simulink model "InteriorPMSMFieldOrientedControl1"  (R2024a)
settings: Solver=FixedStepDiscrete  StartTime=0.0  StopTime=2  RelTol=1e-3  EnableMultiTasking=on
PreLoadFcn:
  | InteriorPMSMFieldOrientedControlData_Lafae
InitFcn:
  | InteriorPMSMFieldOrientedControlData_Lafae
values from neighbouring files (symbols this model uses):
  F = 0.002    [InteriorPMSMFieldOrientedControlData_Lafae.m]
  Fsw = 8000    [InteriorPMSMFieldOrientedControlData_Lafae.m]
  J = 0.09    [InteriorPMSMFieldOrientedControlData_Lafae.m]
  Ki_Ireg = (Ki_Id + Ki_Iq)/2    (= 650)    [InteriorPMSMFieldOrientedControlData_Lafae.m]
  Ki_wreg = (alpha_s/(2*eta))^2*J    [InteriorPMSMFieldOrientedControlData_Lafae.m]
  Kp_Ireg = (Kp_Id + Kp_Iq)/2    (= 182.7)    [InteriorPMSMFieldOrientedControlData_Lafae.m]
  Kp_wreg = alpha_s * J    [InteriorPMSMFieldOrientedControlData_Lafae.m]
  lambda = 0.1757    [InteriorPMSMFieldOrientedControlData_Lafae.m]
  Ld = 1.597e-3    (= 0.001597)    [InteriorPMSMFieldOrientedControlData_Lafae.m]
  Ld_var = 0.9*1.597e-3    (= 0.0014373)    [InteriorPMSMFieldOrientedControlData_Lafae.m]
  Limit_Ireg = Vdc_nom/sqrt(3)    [InteriorPMSMFieldOrientedControlData_Lafae.m]
  Limit_wreg = Tnom    (= 400)    [InteriorPMSMFieldOrientedControlData_Lafae.m]
  Lq = 2.057e-3    (= 0.002057)    [InteriorPMSMFieldOrientedControlData_Lafae.m]
  Lq_var = 0.9*2.057e-3    (= 0.0018513)    [InteriorPMSMFieldOrientedControlData_Lafae.m]
  p = 4    [InteriorPMSMFieldOrientedControlData_Lafae.m]
  rpm_data = [0 1200 2000 3000 4000 5000 6000]    [InteriorPMSMFieldOrientedControlData_Lafae.m]
  Rs = 6.5e-3    (= 0.0065)    [InteriorPMSMFieldOrientedControlData_Lafae.m]
  Tmax_data = [400 400 225 150 100 80 70]    [InteriorPMSMFieldOrientedControlData_Lafae.m]
  Tnom = 400    [InteriorPMSMFieldOrientedControlData_Lafae.m]
  Ts = 10e-6    (= 1e-05)    [InteriorPMSMFieldOrientedControlData_Lafae.m]
  Vdc_nom = 550    [InteriorPMSMFieldOrientedControlData_Lafae.m]
  wmax = 6000    [InteriorPMSMFieldOrientedControlData_Lafae.m]
undefined symbols (not defined in the file or in its folder): DiscIntNeverNeededParam, gcbh, sps_rtmsupport
libraries: simulink x11, spsSecondOrderFilterLib x6, spsStairGeneratorLib x6, spsPermanentMagnetSynchronousMachineLib x1, spsDCVoltageSourceLib x1, spsdq0toabcLib x1, spsabctodq0Lib x1, spsPowerdq0InstantaneousLib x1, spsThreePhaseVIMeasurementLib x1, spsTwoLevelConverterLib x1, spspowerguiLib x1
settings Model: SimulationMode=accelerator  Creator=The MathWorks, Inc.  LastModifiedBy=luansantos
settings SolverCC: AlgebraicLoopSolver=TrustRegion
settings DataIOCC: SaveOutput=off  SignalLogging=off  DSMLogging=off  SaveTime=off  ReturnWorkspaceOutputs=off
settings DebuggingCC: UnconnectedInputMsg=warning  UnconnectedOutputMsg=warning  UnconnectedLineMsg=warning
settings ModelReferenceCC: EnableRefExpFcnMdlSchedulingChecks=on
settings RTWCC: GPUComputeCapability=3.5  DLArmComputeVersion=19.05

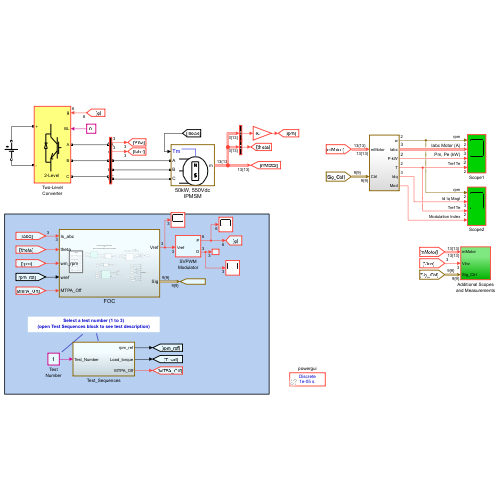
[thumbnail: Simulink's stored preview of the top-level diagram]
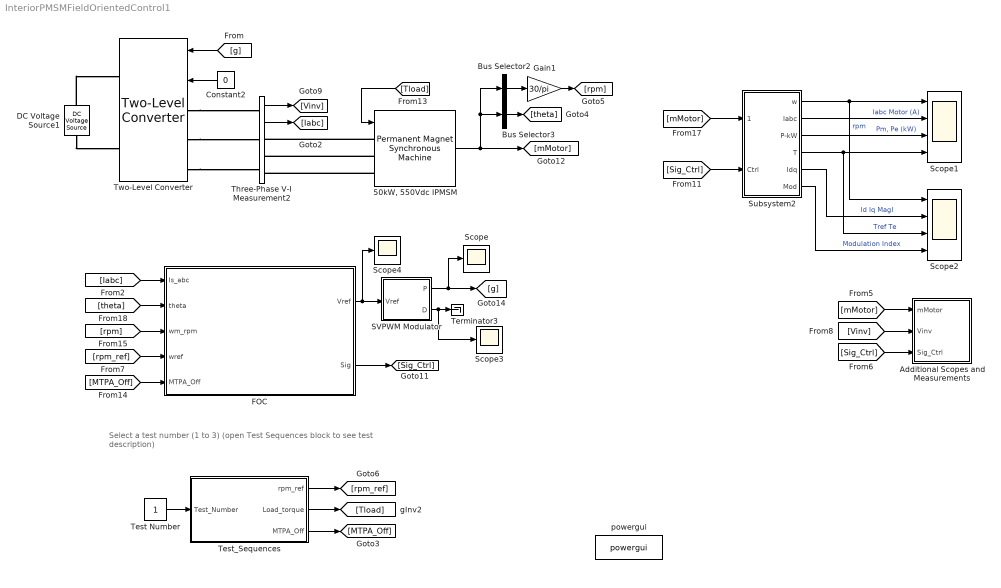
== system InteriorPMSMFieldOrientedControl1 ==
  note: Select a test number (1 to 3)
      | (open Test Sequences block to see test description)
  "50kW, 550Vdc IPMSM" : spsPermanentMagnetSynchronousMachineLib/Permanent Magnet Synchronous Machine  NbPhases=3  FluxDistribution=Sinusoidal  RotorType=Salient-pole  MechanicalLoad=Torque Tm  PresetModel=No  ShowDetailedParameters=on  MeasurementBus=off  Resistance=Rs  Inductance=8.5e-3  dqInductances=[Ld_var, Lq_var]  La=0.005/2  MachineConstant=Flux linkage established by magnets (V.s)  Flux=lambda_var  VoltageCst=127.4738  TorqueCst=1.0542  Flat=120  Mechanical=[J F p 0]  PolePairs=4  InitialConditions=[0,0, 0,0]  InitialConditions5ph=[0 0 0 0 0 0]  RefAngle=90 degrees behind phase A axis (modified Park)  IterativeDiscreteModel=Trapezoidal robust  TsBlock=Ts  TsPowergui=0
  Additional Scopes and Measurements : Subsystem
  Bus Selector2 : BusSelector  OutputSignals=Rotor speed wm (rad/s)  OutputAsBus=on
  Bus Selector3 : BusSelector  OutputSignals=Rotor angle thetam (rad)  OutputAsBus=on
  Constant2 : Constant  Value=0
  DC Voltage Source1 : spsDCVoltageSourceLib/DC Voltage Source  Amplitude=Vdc_nom  Measurements=None
  FOC : Subsystem
  Gain1 : Gain  Gain=30/pi
  SVPWM Modulator : Subsystem  DialogController=POWERSYS.PowerSysDialog  LoadFcn=sps_rtmsupport('LoadFcn', gcbh);  StartFcn=sps_rtmsupport('StartFcn', gcbh);  StopFcn=sps_rtmsupport('StopFcn', gcbh);  mask(Unified PWM Modulator for a 2-level, 3-phase converter){PWMmethod=Space Vector PWM (SVPWM) with pulse averaging, Fsw=Fsw, Ts=Ts}
      mask prompts: PWMmethod "PWM method"; Fsw "Switching frequency (Hz):"; Ts "Sample time (s):"
      mask help:
      | Generate pulses for PWM-controlled two-level, three-phase power electronics converter with pulse averaging capability.
      |
      | The pulses generation can be perform using one of the following Pulse-Width Modulation (PWM) methods:
      | 1. Sinusoidal PWM (SPWM)
      | 2. Sinusoidal PWM (SPWM) with pulse averaging
      | 3. Space Vector PWM (SVPWM)
      | 4. Space Vector PWM (SVPWM) with pulse averaging
      | 5. 30 degrees discontinuous PWM
      |
      | When a PWM method with pulse averaging is selected, the output pulses are averaged over one sample time. (Pulses value will range from 0 to 1)
      mask init:
      | switch PWMmethod
      |     case 1 % SPWM
      |         ZeroOrderHold_Ts=-1;
      |         Pavg=0;
      |     case 2 % SPWM with pulse averaging
      |         ZeroOrderHold_Ts=-1;
      |         Pavg=1;
      |     case 3  % SVPWM
      |         ZeroOrderHold_Ts=-1;
      |         Pavg=0;
      |     case 4  % SVPWM with pulse averaging
      |         ZeroOrderHold_Ts=-1;
      |         Pavg=1;
      |     case 5  % 30 degrees discontinuous PWM
      |         ZeroOrderHold_Ts=1/Fsw/2;
      |         Pavg=0;
      | end
      settings: CopyFcn=sps_rtmsupport('CopyFcn', gcbh);  DeleteFcn=sps_rtmsupport('DeleteFcn', gcbh);  UndoDeleteFcn=sps_rtmsupport('UndoDeleteFcn', gcbh);  ModelCloseFcn=sps_rtmsupport('ModelCloseFcn', gcbh);  PreSaveFcn=sps_rtmsupport('PreSaveFcn', gcbh);  PostSaveFcn=sps_rtmsupport('PostSaveFcn', gcbh);  NameChangeFcn=sps_rtmsupport('NameChangeFcn', gcbh);  PreCopyFcn=sps_rtmsupport('PreCopyFcn', gcbh);  OpenFcn=sps_rtmsupport('OpenFcn', gcbh, [1]);  CloseFcn=sps_rtmsupport('CloseFcn', gcbh);  PreDeleteFcn=sps_rtmsupport('PreDeleteFcn', gcbh);
      mask TypeOptions PWMmethod: Sinusoidal PWM (SPWM) | Sinusoidal PWM (SPWM) wirh pulse averaging | Space Vector PWM (SVPWM) | Space Vector PWM (SVPWM) with pulse averaging | 30 degrees discontinuous PWM
  Scope : Scope
  Scope1 : Scope  NumInputPorts=4
  Scope2 : Scope  NumInputPorts=4
  Scope3 : Scope
  Scope4 : Scope
  Subsystem2 : Subsystem
  Terminator3 : Terminator
  Test Number : Constant
  Test_Sequences : Subsystem
  Three-Phase V-I Measurement2 : spsThreePhaseVIMeasurementLib/Three-Phase V-I Measurement  VoltageMeasurement=phase-to-phase  SetLabelV=off  LabelV=Vabc  Vpu=off  VpuLL=off  CurrentMeasurement=yes  SetLabelI=off  LabelI=Iabc  Ipu=off  Pbase=100e6  Vbase=500e3  OutputType=Complex  PhasorSimulation=off  PSBequivalent=0
  Two-Level Converter : spsTwoLevelConverterLib/Two-Level Converter  ModelType=Switching function  Ron=1e-3  Rs=1e6  Cs=inf  Vforward=[0,0]  Ron_Diode=1e-3  Rs_Diode=1e6  Cs_Diode=inf  Vf_Diode=0  Rs_CurrentSource=inf  Ron_ACsource=1e-3
  powergui : spspowerguiLib/powergui  SimulationMode=Discrete  SampleTime=Ts  frequency=60  Iterations=50  frequencyindice=0  Pbase=100e6  ErrMax=1e-4  UnitsV=kV  UnitsW=MW  buscounter=0  FunctionMessages=off  echomessages=off  EnableUseOfTLC=off  CurrentSourceSwitches=off  DisableSnubberDevices=off  DisableRonSwitches=off  DisableVfSwitches=off  DisplayEquations=off  AutomaticDiscreteSolvers=off  SolverType=Tustin  Interpol=off  ExternalGateDelay=off  methode=off  Ts=0  x0status=blocks  SPID=off  SwTol=0  HookPort=off  NonlinearTolerance=1e-4  nMaxIteration=100  ContinueOnMaxIteration=off  RestoreLinks=warning  ResistiveCurrentMeasurement=off  Frange=[0:2:500]  Ylog=off  Xlog=on  ShowGrid=off  save=off  variable=ZData  structure=ScopeData3  ZoomFFT=off  StartTime=0.95  cycles=1  DisplayStyle=1  fundamental=166.67  FreqAxis=off  MaxFrequency=20000  frequencyindicesteady=1  RmsSteady=1  display=off
  wires:
  [Iabc] -> FOC/1(Is_abc)
  Gain1/1 -> [rpm]
  "50kW, 550Vdc IPMSM"/1 -> [mMotor], Bus Selector3/1, Bus Selector2/1
  Test Number/1 -> Test_Sequences/1(Test_Number)
  Test_Sequences/2(Load_torque) -> [Tload]
  [MTPA_Off] -> FOC/5(MTPA_Off)
  SVPWM Modulator/1(P) -> Scope/1, [g]
  [theta] -> FOC/2(theta)
  Constant2/1 -> Two-Level Converter/2
  FOC/2(Sig) -> [Sig_Ctrl]
  Test_Sequences/1(rpm_ref) -> [rpm_ref]
  [mMotor] -> Subsystem2/1(mMotor)
  [rpm] -> FOC/3(wm_rpm)
  SVPWM Modulator/2(D) -> Scope3/1, Terminator3/1
  Subsystem2/3(P-kW) -> Scope1/3  "Pm, Pe (kW)"
  Bus Selector2/1 -> Gain1/1
  FOC/1(Vref) -> Scope4/1, SVPWM Modulator/1(Vref)
  [rpm_ref] -> FOC/4(wref)
  Three-Phase V-I Measurement2/2 -> [Iabc]
  [Sig_Ctrl] -> Subsystem2/2(Ctrl)
  Three-Phase V-I Measurement2/1 -> [Vinv]
  Bus Selector3/1 -> [theta]
  [g] -> Two-Level Converter/1
  Subsystem2/2(Iabc) -> Scope1/2  "Iabc Motor (A)"
  Test_Sequences/3(MTPA_Off) -> [MTPA_Off]
  Subsystem2/1(w) -> Scope1/1, Scope2/1  "rpm"
  Subsystem2/5(Idq) -> Scope2/2  "Id Iq MagI"
  Subsystem2/4(T) -> Scope1/4, Scope2/3  "Tref Te"
  [Vinv] -> Additional Scopes and Measurements/2(Vinv)
  [mMotor] -> Additional Scopes and Measurements/1(mMotor)
  [Sig_Ctrl] -> Additional Scopes and Measurements/3(Sig_Ctrl)
  Subsystem2/6(Mod) -> Scope2/4  "Modulation Index"
  [Tload] -> "50kW, 550Vdc IPMSM"/1
  connections:
  DC Voltage Source1/LConn1 -- Two-Level Converter/RConn2
  Two-Level Converter/LConn2 -- Three-Phase V-I Measurement2/LConn2
  Two-Level Converter/LConn1 -- Three-Phase V-I Measurement2/LConn1
  DC Voltage Source1/RConn1 -- Two-Level Converter/RConn1
  "50kW, 550Vdc IPMSM"/LConn2 -- Three-Phase V-I Measurement2/RConn2
  Two-Level Converter/LConn3 -- Three-Phase V-I Measurement2/LConn3
  "50kW, 550Vdc IPMSM"/LConn1 -- Three-Phase V-I Measurement2/RConn1
  "50kW, 550Vdc IPMSM"/LConn3 -- Three-Phase V-I Measurement2/RConn3

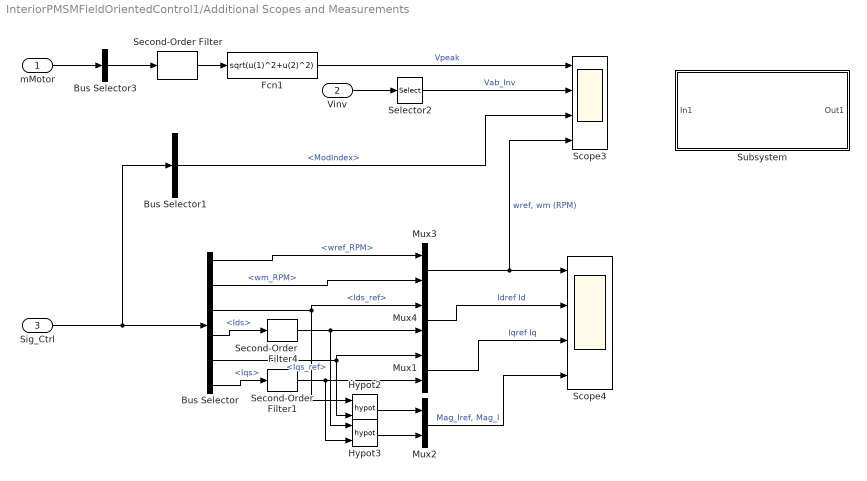
== system InteriorPMSMFieldOrientedControl1/Additional Scopes and Measurements ==
  mMotor : Inport
  Vinv : Inport  Port=2
  Sig_Ctrl : Inport  Port=3
  Bus Selector : BusSelector  OutputSignals=wref_RPM,wm_RPM,Ids_ref,Ids,Iqs_ref,Iqs
  Bus Selector1 : BusSelector  OutputSignals=ModIndex
  Bus Selector3 : BusSelector  OutputSignals=Stator voltage Vs_d (V),Stator voltage Vs_q (V)  OutputAsBus=on
  Fcn1 : Fcn  Expr=sqrt(u(1)^2+u(2)^2)
  Hypot2 : Math  Operator=hypot
  Hypot3 : Math  Operator=hypot
  Mux{1..4} (4 alike) : Mux  Inputs=2
  Scope3 : Scope  NumInputPorts=4
  Scope4 : Scope  NumInputPorts=4
  Second-Order Filter : spsSecondOrderFilterLib/Second-Order Filter  FilterType=Lowpass  Fo=120  Zeta=1  Ts=Ts  Initialize=off  Vac_Init="[0,  0,  60]"  Vdc_Init=0  PlotResponse=off  FreqRange=[0, 500, 1]
  Second-Order Filter1 : spsSecondOrderFilterLib/Second-Order Filter  FilterType=Lowpass  Fo=80  Zeta=1  Ts=Ts  Initialize=off  Vac_Init="[0,  0,  60]"  Vdc_Init=0  PlotResponse=off  FreqRange=[0, 500, 1]
  Second-Order Filter4 : spsSecondOrderFilterLib/Second-Order Filter  FilterType=Lowpass  Fo=80  Zeta=1  Ts=Ts  Initialize=off  Vac_Init="[0,  0,  60]"  Vdc_Init=0  PlotResponse=off  FreqRange=[0, 500, 1]
  Selector2 : Selector  InputPortWidth=3  IndexOptions=Index vector (dialog)  Indices=1  OutputSizes=1
  Subsystem : Subsystem
  wires:
  Bus Selector3/1 -> Second-Order Filter/1
  mMotor/1 -> Bus Selector3/1
  Second-Order Filter/1 -> Fcn1/1
  Bus Selector1/1 -> Scope3/3  "<ModIndex>"
  Mux2/1 -> Scope4/4  "Mag_Iref, Mag_I"
  Mux1/1 -> Scope4/3  "Iqref Iq"
  Mux4/1 -> Scope4/2  "Idref Id"
  Mux3/1 -> Scope4/1, Scope3/4  "wref, wm (RPM)"
  Bus Selector/2 -> Mux3/2  "<wm_RPM>"
  Bus Selector/1 -> Mux3/1  "<wref_RPM>"
  Hypot3/1 -> Mux2/2
  Hypot2/1 -> Mux2/1
  Second-Order Filter1/1 -> Mux1/2, Hypot3/2
  Second-Order Filter4/1 -> Mux4/2, Hypot3/1
  Bus Selector/6 -> Second-Order Filter1/1  "<Iqs>"
  Bus Selector/5 -> Hypot2/2, Mux1/1  "<Iqs_ref>"
  Bus Selector/4 -> Second-Order Filter4/1  "<Ids>"
  Bus Selector/3 -> Hypot2/1, Mux4/1  "<Ids_ref>"
  Sig_Ctrl/1 -> Bus Selector/1, Bus Selector1/1
  Vinv/1 -> Selector2/1
  Fcn1/1 -> Scope3/1  "Vpeak"
  Selector2/1 -> Scope3/2  "Vab_Inv"

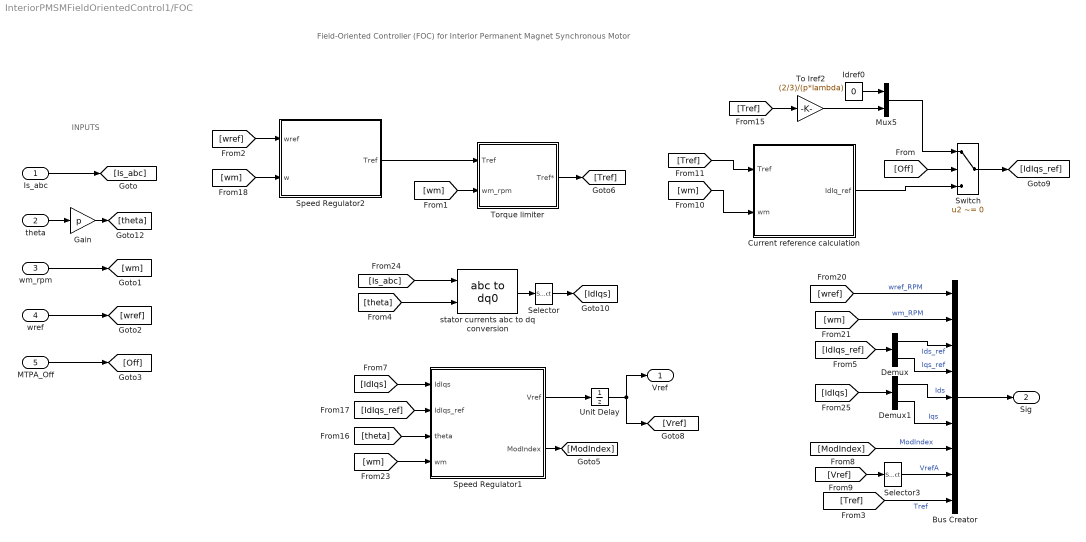
== system InteriorPMSMFieldOrientedControl1/FOC ==
  note: INPUTS
  note: Field-Oriented Controller (FOC)
      | for
      | Interior Permanent Magnet Synchronous Motor
  Is_abc : Inport  PortDimensions=3
  theta : Inport  Port=2  PortDimensions=1
  wm_rpm : Inport  Port=3  PortDimensions=1
  wref : Inport  Port=4  PortDimensions=1
  MTPA_Off : Inport  Port=5  PortDimensions=1
  Bus Creator : BusCreator  Inputs=9
  Current reference calculation : Subsystem  mask(Current reference generation){p=p, LdLq=[Ld, Lq], lambda=lambda, Ts=Ts}
      mask prompts: p "Motor pairs of poles"; LdLq "Inductances [ Ld(H) Lq(H) ]:"; lambda "Flux linkage established by magnets (V.s)"; Ts "Sampling time (s)"
      mask init:
      | Ld=LdLq(1);
      | Lq=LdLq(2);
      | ib = lambda/(Lq-Ld);
      | Teb = 3/2*p*lambda*ib;
      | lam = lambda;
      | ib = lam/(Lq-Ld);
      | iqn = 0:0.01:3;
      | ten = iqn/2.*(sqrt(4*iqn.*iqn+1)+1);
  Demux : Demux  Outputs=2
  Demux1 : Demux  Outputs=2
  Gain : Gain  Gain=p
  Idref0 : Constant  Value=0
  Mux5 : Mux  Inputs=2
  Selector : Selector  InputPortWidth=3  IndexOptions=Index vector (dialog)  Indices=[1 2]  OutputSizes=1
  Selector3 : Selector  InputPortWidth=3  IndexOptions=Index vector (dialog)  Indices=1  OutputSizes=1
  Speed Regulator1 : Subsystem  DialogController=POWERSYS.PowerSysDialog  mask(dq Current Regulators){Kp=Kp_Ireg, Ki=Ki_Ireg, Limits=Limit_Ireg, Init=0, Ts=Ts}
      mask prompts: Kp "Proportional gain (Kp):"; Ki "Integral gain (Ki):"; Limits "Output limits"; Init "Output initial value:"; Ts "Sample time:"
      mask help: This block implements dq currents regulator using anti-windup PI controllers and feedforward calculation.
      mask Display: disp('Current\nRegulators');
  Speed Regulator2 : Subsystem  DialogController=POWERSYS.PowerSysDialog  mask(Speed Regulator){Kp=Kp_wreg, Ki=Ki_wreg, Limit_wreg=Limit_wreg, Init=0, Ts=Ts}
      mask prompts: Kp "Proportional gain (Kp):"; Ki "Integral gain (Ki):"; Limit_wreg "Output limits"; Init "Output initial value:"; Ts "Sample time:"
      mask help: This block implements a speed regulator using an ant-windup PI controller.
      mask Display: disp('Speed\nRegulator');
  Switch : Switch  Criteria=u2 ~= 0  SaturateOnIntegerOverflow=off  InputSameDT=off
  To Iref2 : Gain  Gain=(2/3)/(p*lambda)
  Torque limiter : Subsystem
      mask Display: plot([0;1800;2000;2500;3000;3500], [1;1;0.90*1;0.72*1;0.6*1;0.51*1])
  Unit Delay : UnitDelay  SampleTime=-1  HasFrameUpgradeWarning=on
  stator currents abc to dq conversion : spsabctodq0Lib/abc to dq0  Alignment=90 degrees behind phase A axis
  Vref : Outport  PortDimensions=3
  Sig : Outport  Port=2
  wires:
  [wm] -> Torque limiter/2(wm_rpm)
  Speed Regulator2/1(Tref) -> Torque limiter/1(Tref)
  [Tref] -> To Iref2/1
  Torque limiter/1(Tref*) -> [Tref]
  [wref] -> Speed Regulator2/1(wref)
  To Iref2/1 -> Mux5/2
  [Tref] -> Bus Creator/9  "Tref"
  Speed Regulator1/1(Vref) -> Unit Delay/1
  [Off] -> Switch/2
  MTPA_Off/1 -> [Off]
  wm_rpm/1 -> [wm]
  [ModIndex] -> Bus Creator/7  "ModIndex"
  [IdIqs_ref] -> Demux/1
  Demux/2 -> Bus Creator/4  "Iqs_ref"
  [Is_abc] -> stator currents abc to dq conversion/1
  wref/1 -> [wref]
  stator currents abc to dq conversion/1 -> Selector/1
  Switch/1 -> [IdIqs_ref]
  Selector/1 -> [IdIqs]
  Unit Delay/1 -> Vref/1, [Vref]
  Selector3/1 -> Bus Creator/8  "VrefA"
  Idref0/1 -> Mux5/1
  Mux5/1 -> Switch/1
  [theta] -> stator currents abc to dq conversion/2
  theta/1 -> Gain/1
  [IdIqs] -> Speed Regulator1/1(IdIqs)
  [wm] -> Speed Regulator2/2(w)
  Bus Creator/1 -> Sig/1
  [theta] -> Speed Regulator1/3(theta)
  Demux/1 -> Bus Creator/3  "Ids_ref"
  [wm] -> Bus Creator/2  "wm_RPM"
  [IdIqs_ref] -> Speed Regulator1/2(IdIqs_ref)
  [IdIqs] -> Demux1/1
  [wm] -> Speed Regulator1/4(wm)
  Demux1/2 -> Bus Creator/6  "Iqs"
  [Vref] -> Selector3/1
  Demux1/1 -> Bus Creator/5  "Ids"
  Speed Regulator1/2(ModIndex) -> [ModIndex]
  Is_abc/1 -> [Is_abc]
  [wref] -> Bus Creator/1  "wref_RPM"
  Gain/1 -> [theta]
  [wm] -> Current reference calculation/2(wm)
  [Tref] -> Current reference calculation/1(Tref)
  Current reference calculation/1(IdIq_ref) -> Switch/3

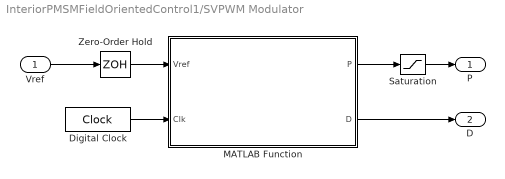
== system InteriorPMSMFieldOrientedControl1/SVPWM Modulator ==
  Vref : Inport  PortDimensions=3  SampleTime=Ts
  Digital Clock : DigitalClock  SampleTime=Ts
  MATLAB Function : MATLAB Function  TreatAsAtomicUnit=on
  Saturation : Saturate  UpperLimit=1  LowerLimit=0
  Zero-Order Hold : ZeroOrderHold  SampleTime=ZeroOrderHold_Ts
  P : Outport  PortDimensions=6  SampleTime=Ts  VectorParamsAs1DForOutWhenUnconnected=off
  D : Outport  Port=2  PortDimensions=3  SampleTime=Ts  VectorParamsAs1DForOutWhenUnconnected=off
  wires:
  Zero-Order Hold/1 -> MATLAB Function/1(Vref)
  Digital Clock/1 -> MATLAB Function/2(Clk)
  Saturation/1 -> P/1
  Vref/1 -> Zero-Order Hold/1
  MATLAB Function/1(P) -> Saturation/1
  MATLAB Function/2(D) -> D/1

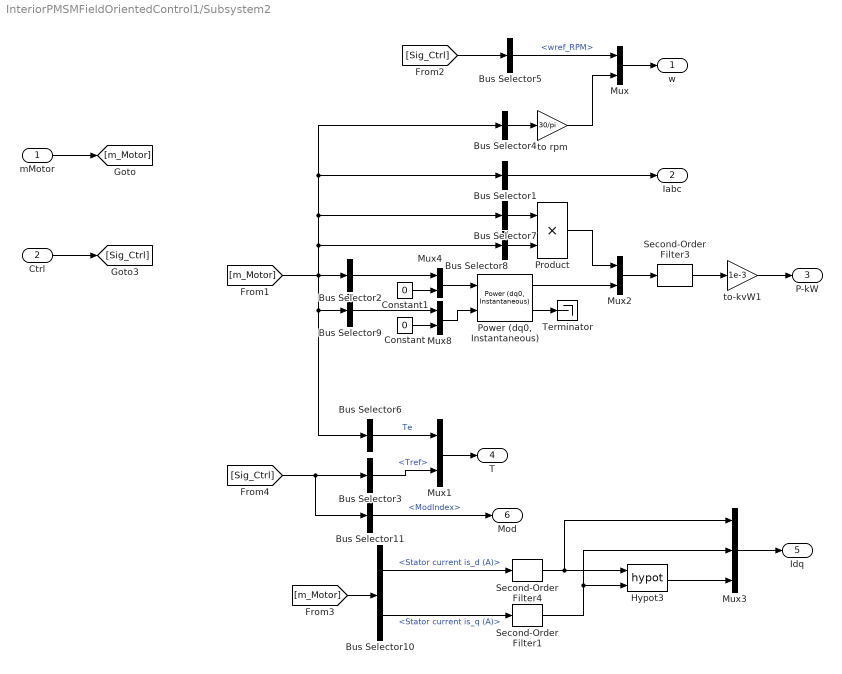
== system InteriorPMSMFieldOrientedControl1/Subsystem2 ==
  mMotor : Inport
  Ctrl : Inport  Port=2
  Bus Selector1 : BusSelector  OutputSignals=Stator current is_a (A),Stator current is_b (A),Stator current is_c (A)  OutputAsBus=on
  Bus Selector10 : BusSelector  OutputSignals=Stator current is_d (A),Stator current is_q (A)
  Bus Selector11 : BusSelector  OutputSignals=ModIndex
  Bus Selector2 : BusSelector  OutputSignals=Stator voltage Vs_d (V),Stator voltage Vs_q (V)  OutputAsBus=on
  Bus Selector3 : BusSelector  OutputSignals=Tref
  Bus Selector4 : BusSelector  OutputSignals=Rotor speed wm (rad/s)  OutputAsBus=on
  Bus Selector5 : BusSelector  OutputSignals=wref_RPM
  Bus Selector6 : BusSelector  OutputSignals=Electromagnetic torque Te (N*m)  OutputAsBus=on
  Bus Selector7 : BusSelector  OutputSignals=Rotor speed wm (rad/s)  OutputAsBus=on
  Bus Selector8 : BusSelector  OutputSignals=Electromagnetic torque Te (N*m)  OutputAsBus=on
  Bus Selector9 : BusSelector  OutputSignals=Stator current is_d (A),Stator current is_q (A)  OutputAsBus=on
  Constant : Constant  Value=0
  Constant1 : Constant  Value=0
  Hypot3 : Math  Operator=hypot
  Mux : Mux  Inputs=2
  Mux1 : Mux  Inputs=2
  Mux2 : Mux  Inputs=2
  Mux3 : Mux  Inputs=3
  Mux4 : Mux  Inputs=[2, 1]
  Mux8 : Mux  Inputs=[2, 1]
  "Power (dq0, Instantaneous)" : spsPowerdq0InstantaneousLib/Power (dq0, Instantaneous)
  Product : Product
  Second-Order Filter1 : spsSecondOrderFilterLib/Second-Order Filter  FilterType=Lowpass  Fo=80  Zeta=1  Ts=Ts  Initialize=off  Vac_Init="[0,  0,  60]"  Vdc_Init=0  PlotResponse=off  FreqRange=[0, 500, 1]
  Second-Order Filter3 : spsSecondOrderFilterLib/Second-Order Filter  FilterType=Lowpass  Fo=80  Zeta=1  Ts=Ts  Initialize=off  Vac_Init="[0,  0,  60]"  Vdc_Init=0  PlotResponse=off  FreqRange=[0, 500, 1]
  Second-Order Filter4 : spsSecondOrderFilterLib/Second-Order Filter  FilterType=Lowpass  Fo=80  Zeta=1  Ts=Ts  Initialize=off  Vac_Init="[0,  0,  60]"  Vdc_Init=0  PlotResponse=off  FreqRange=[0, 500, 1]
  Terminator : Terminator
  to rpm : Gain  Gain=30/pi
  to-kvW1 : Gain  Gain=1e-3
  w : Outport
  Iabc : Outport  Port=2
  P-kW : Outport  Port=3
  T : Outport  Port=4
  Idq : Outport  Port=5
  Mod : Outport  Port=6
  wires:
  Bus Selector1/1 -> Iabc/1
  Mux8/1 -> "Power (dq0, Instantaneous)"/2
  "Power (dq0, Instantaneous)"/1 -> Mux2/2
  Bus Selector2/1 -> Mux4/1
  Constant/1 -> Mux8/2
  Bus Selector9/1 -> Mux8/1
  Constant1/1 -> Mux4/2
  Mux4/1 -> "Power (dq0, Instantaneous)"/1
  [m_Motor] -> Bus Selector6/1, Bus Selector9/1, Bus Selector7/1, Bus Selector4/1, Bus Selector1/1, Bus Selector8/1, Bus Selector2/1
  mMotor/1 -> [m_Motor]
  Mux1/1 -> T/1
  Ctrl/1 -> [Sig_Ctrl]
  [Sig_Ctrl] -> Bus Selector11/1, Bus Selector3/1
  Bus Selector4/1 -> to rpm/1
  Bus Selector5/1 -> Mux/1  "<wref_RPM>"
  [Sig_Ctrl] -> Bus Selector5/1
  to rpm/1 -> Mux/2
  Mux/1 -> w/1
  "Power (dq0, Instantaneous)"/2 -> Terminator/1
  Mux2/1 -> Second-Order Filter3/1
  to-kvW1/1 -> P-kW/1
  Second-Order Filter3/1 -> to-kvW1/1
  Bus Selector7/1 -> Product/1
  Bus Selector8/1 -> Product/2
  Product/1 -> Mux2/1
  Second-Order Filter1/1 -> Mux3/2, Hypot3/2
  Hypot3/1 -> Mux3/3
  Mux3/1 -> Idq/1
  Second-Order Filter4/1 -> Mux3/1, Hypot3/1
  [m_Motor] -> Bus Selector10/1
  Bus Selector10/1 -> Second-Order Filter4/1  "<Stator current is_d (A)>"
  Bus Selector10/2 -> Second-Order Filter1/1  "<Stator current is_q (A)>"
  Bus Selector11/1 -> Mod/1  "<ModIndex>"
  Bus Selector6/1 -> Mux1/1  "Te"
  Bus Selector3/1 -> Mux1/2  "<Tref>"

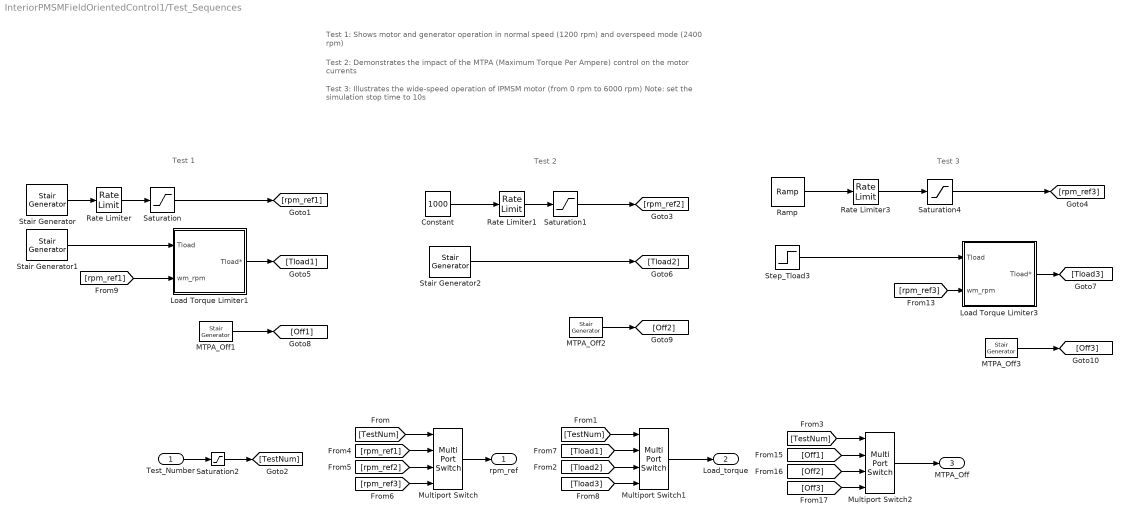
== system InteriorPMSMFieldOrientedControl1/Test_Sequences ==
  note: Test 1
  note: Test 2
  note: Test 3
  note: Test 1: Shows motor and generator operation in normal speed (1200 rpm) and overspeed mode (2400 rpm)
  note: Test 2: Demonstrates the impact of the MTPA (Maximum Torque Per Ampere) control on the motor currents
  note: Test 3: Illustrates the wide-speed operation of IPMSM motor (from 0 rpm to 6000 rpm)
      | Note: set the simulation stop time to 10s
  Test_Number : Inport
  Constant : Constant  Value=1000
  Load Torque Limiter1 : Subsystem
  Load Torque Limiter3 : Subsystem
  MTPA_Off1 : spsStairGeneratorLib/Stair Generator  t=[0, 0.9]  e=[0, 1]*0  Ts=Ts
  MTPA_Off2 : spsStairGeneratorLib/Stair Generator  t=[0, 0.8]  e=[0, 1]  Ts=Ts
  MTPA_Off3 : spsStairGeneratorLib/Stair Generator  t=[0, 1.8]  e=[0, 1]*0  Ts=Ts
  Multiport Switch : MultiPortSwitch  SaturateOnIntegerOverflow=off  InputSameDT=off
  Multiport Switch1 : MultiPortSwitch  SaturateOnIntegerOverflow=off  InputSameDT=off
  Multiport Switch2 : MultiPortSwitch  SaturateOnIntegerOverflow=off  InputSameDT=off
  Ramp : simulink/Sources/Ramp  slope=1000*0.7  start=0.5  InitialOutput=0
  Rate Limiter : RateLimiter  RisingSlewLimit=12000  FallingSlewLimit=-12000  SampleTimeMode=inherited
  Rate Limiter1 : RateLimiter  RisingSlewLimit=10000  FallingSlewLimit=-10000  SampleTimeMode=inherited
  Rate Limiter3 : RateLimiter  RisingSlewLimit=5000  FallingSlewLimit=-5000  SampleTimeMode=inherited
  Saturation : Saturate  UpperLimit=wmax  LowerLimit=0
  Saturation1 : Saturate  UpperLimit=wmax  LowerLimit=0
  Saturation2 : Saturate  UpperLimit=3  LowerLimit=1
  Saturation4 : Saturate  UpperLimit=wmax  LowerLimit=0
  Stair Generator : spsStairGeneratorLib/Stair Generator  t=[0]  e=[1200]  Ts=Ts
  Stair Generator1 : spsStairGeneratorLib/Stair Generator  t=[0,0.4]  e=[0, 350]  Ts=Ts
  Stair Generator2 : spsStairGeneratorLib/Stair Generator  t=[0,0.4]  e=[0, 350 ]  Ts=Ts
  Step_Tload3 : Step  Before=1  After=Tnom  SampleTime=Ts
  rpm_ref : Outport
  Load_torque : Outport  Port=2
  MTPA_Off : Outport  Port=3
  wires:
  Stair Generator/1 -> Rate Limiter/1
  Rate Limiter/1 -> Saturation/1
  Saturation/1 -> [rpm_ref1]
  Multiport Switch/1 -> rpm_ref/1
  Test_Number/1 -> Saturation2/1
  Saturation2/1 -> [TestNum]
  [TestNum] -> Multiport Switch/1
  Rate Limiter3/1 -> Saturation4/1
  Saturation4/1 -> [rpm_ref3]
  [rpm_ref1] -> Multiport Switch/2
  [rpm_ref2] -> Multiport Switch/3
  [rpm_ref3] -> Multiport Switch/4
  [Tload3] -> Multiport Switch1/4
  [Tload2] -> Multiport Switch1/3
  [Tload1] -> Multiport Switch1/2
  [TestNum] -> Multiport Switch1/1
  Multiport Switch1/1 -> Load_torque/1
  Load Torque Limiter3/1(Tload*) -> [Tload3]
  Multiport Switch2/1 -> MTPA_Off/1
  [TestNum] -> Multiport Switch2/1
  [Off1] -> Multiport Switch2/2
  [Off2] -> Multiport Switch2/3
  [Off3] -> Multiport Switch2/4
  MTPA_Off1/1 -> [Off1]
  MTPA_Off2/1 -> [Off2]
  MTPA_Off3/1 -> [Off3]
  Saturation1/1 -> [rpm_ref2]
  Rate Limiter1/1 -> Saturation1/1
  Constant/1 -> Rate Limiter1/1
  Ramp/1 -> Rate Limiter3/1
  [rpm_ref3] -> Load Torque Limiter3/2(wm_rpm)
  [rpm_ref1] -> Load Torque Limiter1/2(wm_rpm)
  Load Torque Limiter1/1(Tload*) -> [Tload1]
  Step_Tload3/1 -> Load Torque Limiter3/1(Tload)
  Stair Generator1/1 -> Load Torque Limiter1/1(Tload)
  Stair Generator2/1 -> [Tload2]

== system InteriorPMSMFieldOrientedControl1/Additional Scopes and Measurements/Subsystem ==
  In1 : Inport
  Out1 : Outport
  wires:
  In1/1 -> Out1/1

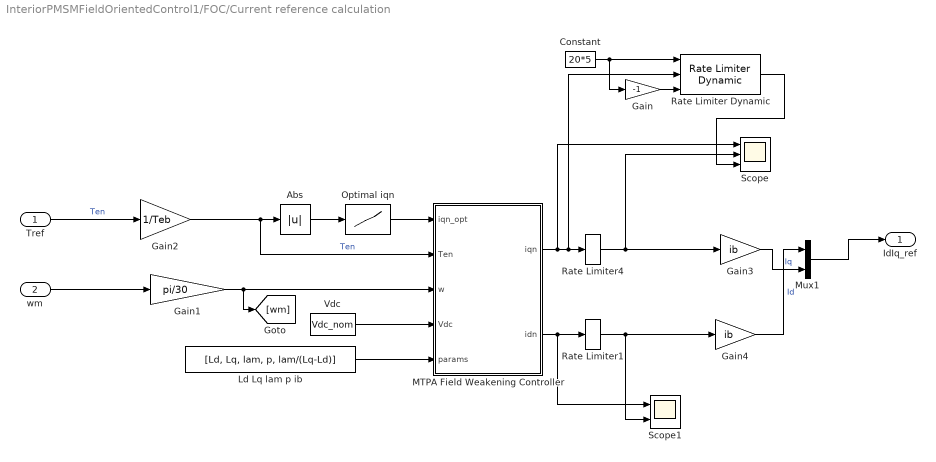
== system InteriorPMSMFieldOrientedControl1/FOC/Current reference calculation ==
  Tref : Inport
  wm : Inport  Port=2
  Abs : Abs  SaturateOnIntegerOverflow=off
  Constant : Constant  Value=20*5
  Gain : Gain  Gain=-1
  Gain1 : Gain  Gain=pi/30
  Gain2 : Gain  Gain=1/Teb  SaturateOnIntegerOverflow=on  OutDataTypeStr=Inherit: Same as input  ParamDataTypeStr=Inherit: Same as input
  Gain3 : Gain  Gain=ib  SaturateOnIntegerOverflow=on  OutDataTypeStr=Inherit: Same as input  ParamDataTypeStr=Inherit: Same as input
  Gain4 : Gain  Gain=ib  SaturateOnIntegerOverflow=on  OutDataTypeStr=Inherit: Same as input  ParamDataTypeStr=Inherit: Same as input
  Ld Lq lam p ib : Constant  Value=[Ld, Lq, lam, p, lam/(Lq-Ld)]
  MTPA Field Weakening Controller : MATLAB Function  TreatAsAtomicUnit=on  SystemSampleTime=Ts
  Mux1 : Mux  Inputs=2
  Optimal iqn : Lookup  InputValues=ten  Table=iqn  SaturateOnIntegerOverflow=off
  Rate Limiter Dynamic : simulink/Discontinuities/Rate Limiter Dynamic
  Rate Limiter1 : RateLimiter  RisingSlewLimit=20  FallingSlewLimit=-20  SampleTimeMode=inherited
  Rate Limiter4 : RateLimiter  RisingSlewLimit=20*5  FallingSlewLimit=-20*5  SampleTimeMode=inherited
  Scope : Scope  NumInputPorts=3
  Scope1 : Scope  NumInputPorts=2
  Vdc : Constant  Value=Vdc_nom
  IdIq_ref : Outport
  wires:
  Gain2/1 -> Abs/1, MTPA Field Weakening Controller/2(Ten)  "Ten"
  wm/1 -> Gain1/1
  Ld Lq lam p ib/1 -> MTPA Field Weakening Controller/5(params)
  Optimal iqn/1 -> MTPA Field Weakening Controller/1(iqn_opt)
  Abs/1 -> Optimal iqn/1
  Vdc/1 -> MTPA Field Weakening Controller/4(Vdc)
  Gain1/1 -> [wm], MTPA Field Weakening Controller/3(w)
  Rate Limiter4/1 -> Scope/2, Gain3/1
  Gain4/1 -> Mux1/1  "Id"
  Gain3/1 -> Mux1/2  "Iq"
  Tref/1 -> Gain2/1  "Ten"
  Mux1/1 -> IdIq_ref/1
  MTPA Field Weakening Controller/2(idn) -> Scope1/1, Rate Limiter1/1
  Rate Limiter1/1 -> Scope1/2, Gain4/1
  Gain/1 -> Rate Limiter Dynamic/3
  Constant/1 -> Gain/1, Rate Limiter Dynamic/1
  MTPA Field Weakening Controller/1(iqn) -> Scope/1, Rate Limiter Dynamic/2, Rate Limiter4/1
  Rate Limiter Dynamic/1 -> Scope/3

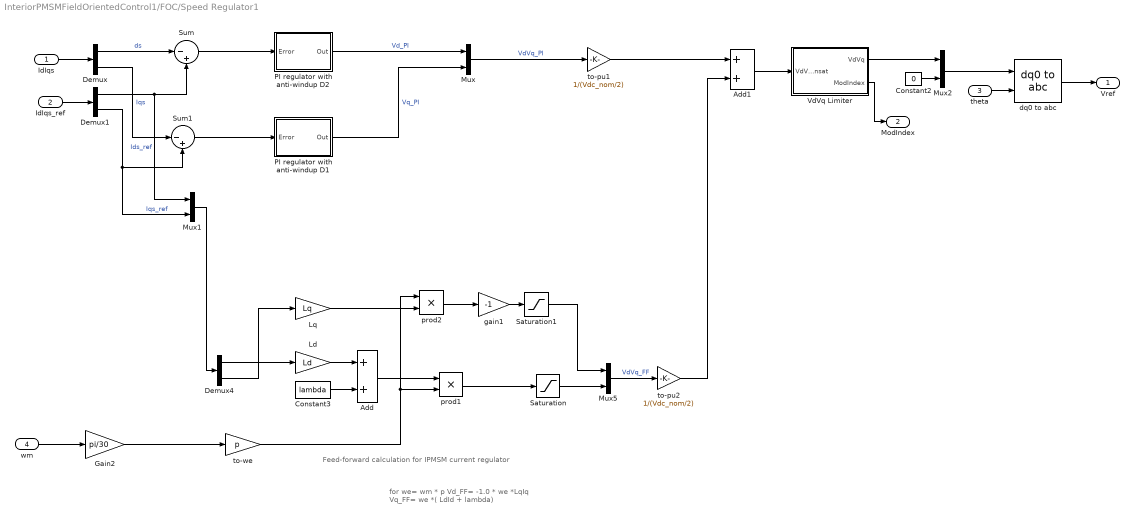
== system InteriorPMSMFieldOrientedControl1/FOC/Speed Regulator1 ==
  note: for we= wm * p
      | Vd_FF= -1.0 * we *LqIq
      | Vq_FF= we *( LdId + lambda)
  note: Feed-forward calculation for IPMSM current regulator
  IdIqs : Inport  PortDimensions=2
  IdIqs_ref : Inport  Port=2  PortDimensions=2
  theta : Inport  Port=3  PortDimensions=1
  wm : Inport  Port=4  PortDimensions=1
  Add : Sum
  Add1 : Sum
  Constant2 : Constant  Value=0
  Constant3 : Constant  Value=lambda  OutDataTypeStr=Inherit: Inherit via back propagation  SampleTime=-1
  Demux : Demux  Outputs=2
  Demux1 : Demux  Outputs=2
  Demux4 : Demux  Outputs=2
  Gain2 : Gain  Gain=pi/30
  Ld : Gain  Gain=Ld  RndMeth=Simplest  OutDataTypeStr=Inherit: Same as input  ParamDataTypeStr=Inherit: Same as input
  Lq : Gain  Gain=Lq  RndMeth=Simplest  OutDataTypeStr=Inherit: Same as input  ParamDataTypeStr=Inherit: Same as input
  Mux : Mux  Inputs=2
  Mux1 : Mux  Inputs=2
  Mux2 : Mux  Inputs=[2,1]
  Mux5 : Mux  Inputs=2
  PI regulator with anti-windup D1 : Subsystem  DialogController=POWERSYS.PowerSysDialog  mask(Discrete PI Controller){Kp=Kp, Ki=Ki, Par_Limits=[Limits -Limits], Init=0, Ts=Ts}
      mask prompts: Kp "Proportional gain (Kp):"; Ki "Integral gain (Ki):"; Par_Limits "Output limits: [ Upper   Lower ]"; Init "Output initial value:"; Ts "Sample time:"
      mask help: This block implements a discrete PI controller.
      mask init:
      | UpperLimit=Par_Limits(1);
      | LowerLimit=Par_Limits(2);
      | power_initmask();
      mask Help: This block is part of a subset of blocks in the Extras library that does not have documentation associated with it, other than the block mask description.
      mask Display: disp('PI');
  PI regulator with anti-windup D2 : Subsystem  DialogController=POWERSYS.PowerSysDialog  mask(Discrete PI Controller){Kp=Kp, Ki=Ki, Par_Limits=[Limits -Limits], Init=0, Ts=Ts}
      mask prompts: Kp "Proportional gain (Kp):"; Ki "Integral gain (Ki):"; Par_Limits "Output limits: [ Upper   Lower ]"; Init "Output initial value:"; Ts "Sample time:"
      mask help: This block implements a discrete PI controller.
      mask init:
      | UpperLimit=Par_Limits(1);
      | LowerLimit=Par_Limits(2);
      | power_initmask();
      mask Help: This block is part of a subset of blocks in the Extras library that does not have documentation associated with it, other than the block mask description.
      mask Display: disp('PI');
  Saturation : Saturate  UpperLimit=Vdc_nom/sqrt(3)  LowerLimit=-Vdc_nom/sqrt(3)  RndMeth=Simplest
  Saturation1 : Saturate  UpperLimit=Vdc_nom/sqrt(3)  LowerLimit=-Vdc_nom/sqrt(3)  RndMeth=Simplest
  Sum : Sum  Inputs=|-+
  Sum1 : Sum  Inputs=|-+
  VdVq Limiter : Subsystem
  dq0 to abc : spsdq0toabcLib/dq0 to abc  Alignment=90 degrees behind phase A axis
  gain1 : Gain  Gain=-1  RndMeth=Simplest  OutDataTypeStr=Inherit: Same as input  ParamDataTypeStr=Inherit: Same as input
  prod1 : Product  RndMeth=Simplest  OutDataTypeStr=Inherit: Same as first input
  prod2 : Product  RndMeth=Simplest  OutDataTypeStr=Inherit: Same as first input
  to-pu1 : Gain  Gain=1/(Vdc_nom/2)
  to-pu2 : Gain  Gain=1/(Vdc_nom/2)
  to-we : Gain  Gain=p  RndMeth=Simplest  OutDataTypeStr=Inherit: Same as input  ParamDataTypeStr=Inherit: Same as input
  Vref : Outport
  ModIndex : Outport  Port=2
  wires:
  to-pu2/1 -> Add1/2
  to-pu1/1 -> Add1/1
  Demux1/1 -> Mux1/1, Sum/2  "Ids_ref"
  Demux/1 -> Sum/1  "ds"
  Demux1/2 -> Sum1/2, Mux1/2  "Iqs_ref"
  IdIqs_ref/1 -> Demux1/1
  IdIqs/1 -> Demux/1
  Sum/1 -> PI regulator with anti-windup D2/1(Error)
  Sum1/1 -> PI regulator with anti-windup D1/1(Error)
  theta/1 -> dq0 to abc/2
  Demux/2 -> Sum1/1  "Iqs"
  dq0 to abc/1 -> Vref/1
  wm/1 -> Gain2/1
  Mux1/1 -> Demux4/1
  PI regulator with anti-windup D2/1(Out) -> Mux/1  "Vd_PI"
  PI regulator with anti-windup D1/1(Out) -> Mux/2  "Vq_PI"
  Mux/1 -> to-pu1/1  "VdVq_PI"
  Mux5/1 -> to-pu2/1  "VdVq_FF"
  Add1/1 -> VdVq Limiter/1(VdVq_unsat)
  VdVq Limiter/1(VdVq) -> Mux2/1
  Constant2/1 -> Mux2/2
  Mux2/1 -> dq0 to abc/1
  VdVq Limiter/2(ModIndex) -> ModIndex/1
  Demux4/2 -> Lq/1
  Lq/1 -> prod2/2
  gain1/1 -> Saturation1/1
  Demux4/1 -> Ld/1
  Add/1 -> prod1/1
  to-we/1 -> prod2/1, prod1/2
  Saturation1/1 -> Mux5/1
  prod2/1 -> gain1/1
  Constant3/1 -> Add/2
  Saturation/1 -> Mux5/2
  Ld/1 -> Add/1
  prod1/1 -> Saturation/1
  Gain2/1 -> to-we/1

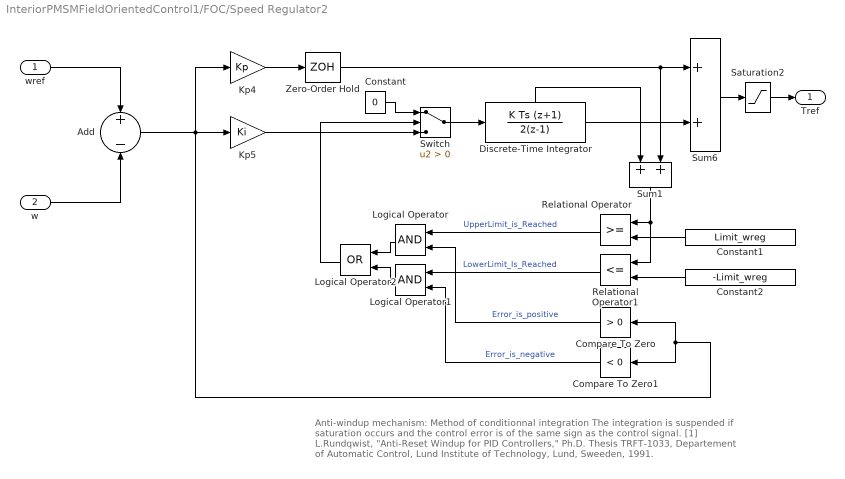
== system InteriorPMSMFieldOrientedControl1/FOC/Speed Regulator2 ==
  note: Anti-windup mechanism: Method of conditionnal integration
      |
      | The integration is suspended if saturation occurs and the
      | control error is of the same sign as the control signal.
      |
      | [1] L.Rundqwist, "Anti-Reset Windup for PID Controllers," Ph.D. Thesis TRFT-1033,
      | Departement of Automatic Control, Lund Institute of Technology, Lund, Sweeden, 1991.
  wref : Inport  PortDimensions=1
  w : Inport  Port=2  PortDimensions=1
  Add : Sum  Inputs=+|-
  Compare To Zero : simulink/Logic and Bit Operations/Compare To Zero  relop=>  OutDataTypeStr=uint8  ZeroCross=off
  Compare To Zero1 : simulink/Logic and Bit Operations/Compare To Zero  relop=<  OutDataTypeStr=uint8  ZeroCross=off
  Constant : Constant  Value=0
  Constant1 : Constant  Value=Limit_wreg
  Constant2 : Constant  Value=-Limit_wreg
  Discrete-Time Integrator : DiscreteIntegrator  IntegratorMethod=Integration: Trapezoidal  InitialCondition=Init  SampleTime=Ts  LimitOutput=on  UpperSaturationLimit=Limit_wreg  LowerSaturationLimit=-Limit_wreg  ShowStatePort=on  ICPrevOutput=DiscIntNeverNeededParam  ICPrevScaledInput=DiscIntNeverNeededParam
  Kp4 : Gain  Gain=Kp  SaturateOnIntegerOverflow=on  SampleTime=Ts  OutDataTypeStr=Inherit: Same as input  ParamDataTypeStr=Inherit: Same as input
  Kp5 : Gain  Gain=Ki  SaturateOnIntegerOverflow=on  SampleTime=Ts  OutDataTypeStr=Inherit: Same as input  ParamDataTypeStr=Inherit: Same as input
  Logical Operator : Logic  AllPortsSameDT=off  OutDataTypeStr=boolean
  Logical Operator1 : Logic  AllPortsSameDT=off  OutDataTypeStr=boolean
  Logical Operator2 : Logic  Operator=OR  AllPortsSameDT=off  OutDataTypeStr=boolean
  Relational Operator : RelationalOperator  OutDataTypeStr=boolean  InputSameDT=off
  Relational Operator1 : RelationalOperator  Operator=<=  OutDataTypeStr=boolean  InputSameDT=off
  Saturation2 : Saturate  UpperLimit=Limit_wreg  LowerLimit=-Limit_wreg  SampleTime=Ts
  Sum1 : Sum  InputSameDT=on  SaturateOnIntegerOverflow=on  SampleTime=Ts  OutDataTypeStr=Inherit: Same as first input
  Sum6 : Sum  InputSameDT=on  SaturateOnIntegerOverflow=on  SampleTime=Ts  OutDataTypeStr=Inherit: Same as first input
  Switch : Switch  Criteria=u2 > Threshold  SaturateOnIntegerOverflow=off  InputSameDT=off
  Zero-Order Hold : ZeroOrderHold  SampleTime=Ts
  Tref : Outport  SampleTime=Ts  InitialOutput=0  VectorParamsAs1DForOutWhenUnconnected=off
  wires:
  w/1 -> Add/2
  wref/1 -> Add/1
  Constant/1 -> Switch/1
  Zero-Order Hold/1 -> Sum1/2, Sum6/1
  Discrete-Time Integrator/State -> Sum1/1
  Sum1/1 -> Relational Operator1/1, Relational Operator/1
  Logical Operator2/1 -> Switch/2
  Relational Operator/1 -> Logical Operator/1  "UpperLimit_is_Reached"
  Relational Operator1/1 -> Logical Operator1/1  "LowerLimit_Is_Reached"
  Constant1/1 -> Relational Operator/2
  Constant2/1 -> Relational Operator1/2
  Compare To Zero/1 -> Logical Operator/2  "Error_is_positive"
  Logical Operator/1 -> Logical Operator2/1
  Logical Operator1/1 -> Logical Operator2/2
  Compare To Zero1/1 -> Logical Operator1/2  "Error_is_negative"
  Add/1 -> Kp4/1, Kp5/1, Compare To Zero1/1, Compare To Zero/1
  Sum6/1 -> Saturation2/1
  Kp4/1 -> Zero-Order Hold/1
  Discrete-Time Integrator/1 -> Sum6/2
  Saturation2/1 -> Tref/1
  Switch/1 -> Discrete-Time Integrator/1
  Kp5/1 -> Switch/3

== system InteriorPMSMFieldOrientedControl1/FOC/Torque limiter ==
  Tref : Inport
  wm_rpm : Inport  Port=2
  Abs1 : Abs
  Gain : Gain  Gain=-1
  Saturation Dynamic : simulink/Discontinuities/Saturation Dynamic  OutMin=[]  OutMax=[]  OutDataTypeStr=Inherit: Same as second input  OutDataType=fixdt(1, 16)  OutScaling=2^-10  DoSatur=off
  Torque vs speed profile1 : Lookup  InputValues=rpm_data  Table=Tmax_data  SaturateOnIntegerOverflow=off
  Tref* : Outport  VectorParamsAs1DForOutWhenUnconnected=off
  wires:
  wm_rpm/1 -> Abs1/1
  Abs1/1 -> Torque vs speed profile1/1
  Torque vs speed profile1/1 -> Saturation Dynamic/1, Gain/1
  Saturation Dynamic/1 -> Tref*/1
  Tref/1 -> Saturation Dynamic/2
  Gain/1 -> Saturation Dynamic/3

== system InteriorPMSMFieldOrientedControl1/Test_Sequences/Load Torque Limiter1 ==
  Tload : Inport
  wm_rpm : Inport  Port=2
  Abs1 : Abs
  Gain : Gain  Gain=-1
  Saturation Dynamic : simulink/Discontinuities/Saturation Dynamic  OutMin=[]  OutMax=[]  OutDataTypeStr=Inherit: Same as second input  OutDataType=fixdt(1, 16)  OutScaling=2^-10  DoSatur=off
  Torque vs speed profile : Lookup_n-D  NumberOfTableDimensions=1  BreakpointsForDimension1=rpm_data  BeginIndexSearchUsingPreviousIndexResult=on  Table=Tmax_data*0.85  InternalRulePriority=Speed
  Tload* : Outport  VectorParamsAs1DForOutWhenUnconnected=off
  wires:
  wm_rpm/1 -> Abs1/1
  Abs1/1 -> Torque vs speed profile/1
  Torque vs speed profile/1 -> Saturation Dynamic/1, Gain/1
  Saturation Dynamic/1 -> Tload*/1
  Tload/1 -> Saturation Dynamic/2
  Gain/1 -> Saturation Dynamic/3

== system InteriorPMSMFieldOrientedControl1/Test_Sequences/Load Torque Limiter3 ==
  Tload : Inport
  wm_rpm : Inport  Port=2
  Abs1 : Abs
  Gain : Gain  Gain=-1
  Saturation Dynamic : simulink/Discontinuities/Saturation Dynamic  OutMin=[]  OutMax=[]  OutDataTypeStr=Inherit: Same as second input  OutDataType=fixdt(1, 16)  OutScaling=2^-10  DoSatur=off
  Torque vs speed profile : Lookup_n-D  NumberOfTableDimensions=1  BreakpointsForDimension1=rpm_data  BeginIndexSearchUsingPreviousIndexResult=on  Table=Tmax_data*0.9  InternalRulePriority=Speed
  Tload* : Outport  VectorParamsAs1DForOutWhenUnconnected=off
  wires:
  Gain/1 -> Saturation Dynamic/3
  Tload/1 -> Saturation Dynamic/2
  Saturation Dynamic/1 -> Tload*/1
  Torque vs speed profile/1 -> Gain/1, Saturation Dynamic/1
  Abs1/1 -> Torque vs speed profile/1
  wm_rpm/1 -> Abs1/1

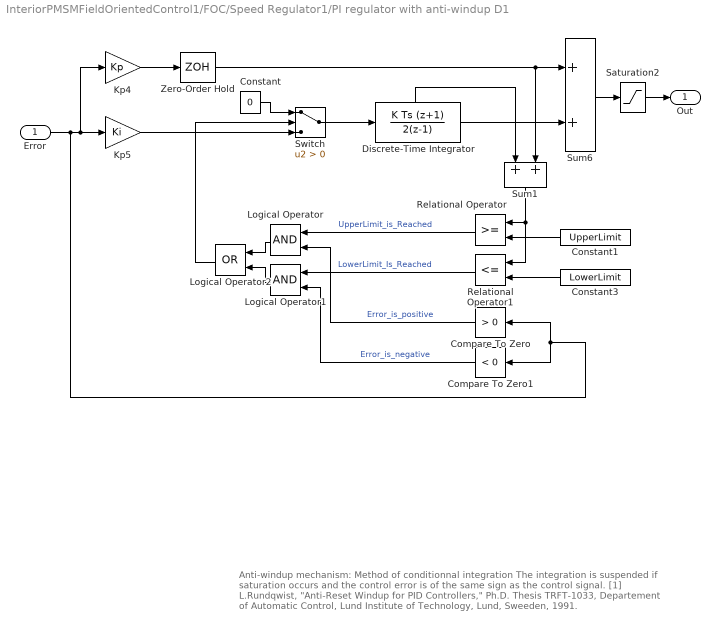
== system InteriorPMSMFieldOrientedControl1/FOC/Speed Regulator1/PI regulator with anti-windup D1 ==
  note: Anti-windup mechanism: Method of conditionnal integration
      |
      | The integration is suspended if saturation occurs and the
      | control error is of the same sign as the control signal.
      |
      | [1] L.Rundqwist, "Anti-Reset Windup for PID Controllers," Ph.D. Thesis TRFT-1033,
      | Departement of Automatic Control, Lund Institute of Technology, Lund, Sweeden, 1991.
  Error : Inport  SampleTime=Ts
  Compare To Zero : simulink/Logic and Bit Operations/Compare To Zero  relop=>  OutDataTypeStr=uint8  ZeroCross=off
  Compare To Zero1 : simulink/Logic and Bit Operations/Compare To Zero  relop=<  OutDataTypeStr=uint8  ZeroCross=off
  Constant : Constant  Value=0
  Constant1 : Constant  Value=UpperLimit
  Constant3 : Constant  Value=LowerLimit
  Discrete-Time Integrator : DiscreteIntegrator  IntegratorMethod=Integration: Trapezoidal  InitialCondition=Init  SampleTime=Ts  LimitOutput=on  UpperSaturationLimit=UpperLimit  LowerSaturationLimit=LowerLimit  ShowStatePort=on  ICPrevOutput=DiscIntNeverNeededParam  ICPrevScaledInput=DiscIntNeverNeededParam
  Kp4 : Gain  Gain=Kp  SaturateOnIntegerOverflow=on  SampleTime=Ts  OutDataTypeStr=Inherit: Same as input  ParamDataTypeStr=Inherit: Same as input
  Kp5 : Gain  Gain=Ki  SaturateOnIntegerOverflow=on  SampleTime=Ts  OutDataTypeStr=Inherit: Same as input  ParamDataTypeStr=Inherit: Same as input
  Logical Operator : Logic  AllPortsSameDT=off  OutDataTypeStr=boolean
  Logical Operator1 : Logic  AllPortsSameDT=off  OutDataTypeStr=boolean
  Logical Operator2 : Logic  Operator=OR  AllPortsSameDT=off  OutDataTypeStr=boolean
  Relational Operator : RelationalOperator  OutDataTypeStr=boolean  InputSameDT=off
  Relational Operator1 : RelationalOperator  Operator=<=  OutDataTypeStr=boolean  InputSameDT=off
  Saturation2 : Saturate  UpperLimit=UpperLimit  LowerLimit=LowerLimit  SampleTime=Ts
  Sum1 : Sum  InputSameDT=on  SaturateOnIntegerOverflow=on  SampleTime=Ts  OutDataTypeStr=Inherit: Same as first input
  Sum6 : Sum  InputSameDT=on  SaturateOnIntegerOverflow=on  SampleTime=Ts  OutDataTypeStr=Inherit: Same as first input
  Switch : Switch  Criteria=u2 > Threshold  SaturateOnIntegerOverflow=off  InputSameDT=off
  Zero-Order Hold : ZeroOrderHold  SampleTime=Ts
  Out : Outport  SampleTime=Ts  InitialOutput=0
  wires:
  Constant/1 -> Switch/1
  Zero-Order Hold/1 -> Sum1/2, Sum6/1
  Discrete-Time Integrator/State -> Sum1/1
  Sum1/1 -> Relational Operator1/1, Relational Operator/1
  Logical Operator2/1 -> Switch/2
  Relational Operator/1 -> Logical Operator/1  "UpperLimit_is_Reached"
  Relational Operator1/1 -> Logical Operator1/1  "LowerLimit_Is_Reached"
  Constant1/1 -> Relational Operator/2
  Constant3/1 -> Relational Operator1/2
  Compare To Zero/1 -> Logical Operator/2  "Error_is_positive"
  Logical Operator/1 -> Logical Operator2/1
  Logical Operator1/1 -> Logical Operator2/2
  Compare To Zero1/1 -> Logical Operator1/2  "Error_is_negative"
  Error/1 -> Compare To Zero1/1, Compare To Zero/1, Kp4/1, Kp5/1
  Sum6/1 -> Saturation2/1
  Kp4/1 -> Zero-Order Hold/1
  Discrete-Time Integrator/1 -> Sum6/2
  Saturation2/1 -> Out/1
  Switch/1 -> Discrete-Time Integrator/1
  Kp5/1 -> Switch/3

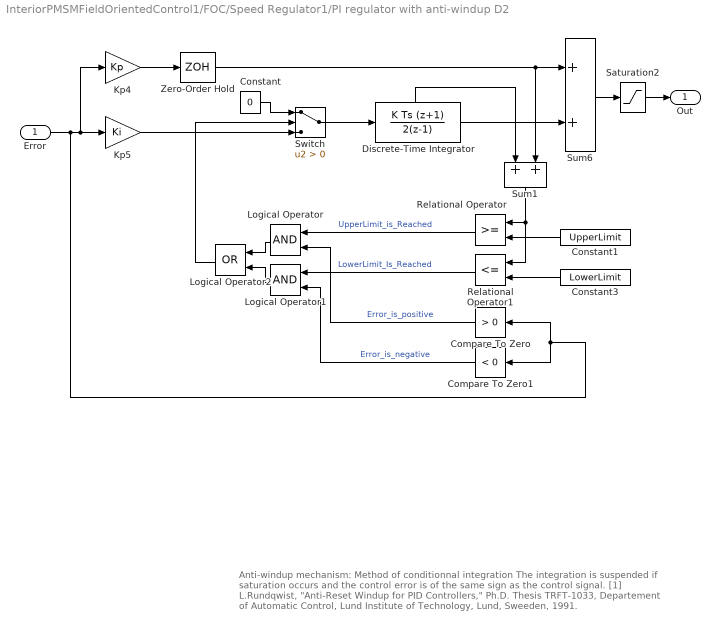
== system InteriorPMSMFieldOrientedControl1/FOC/Speed Regulator1/PI regulator with anti-windup D2 ==
  note: Anti-windup mechanism: Method of conditionnal integration
      |
      | The integration is suspended if saturation occurs and the
      | control error is of the same sign as the control signal.
      |
      | [1] L.Rundqwist, "Anti-Reset Windup for PID Controllers," Ph.D. Thesis TRFT-1033,
      | Departement of Automatic Control, Lund Institute of Technology, Lund, Sweeden, 1991.
  Error : Inport  SampleTime=Ts
  Compare To Zero : simulink/Logic and Bit Operations/Compare To Zero  relop=>  OutDataTypeStr=uint8  ZeroCross=off
  Compare To Zero1 : simulink/Logic and Bit Operations/Compare To Zero  relop=<  OutDataTypeStr=uint8  ZeroCross=off
  Constant : Constant  Value=0
  Constant1 : Constant  Value=UpperLimit
  Constant3 : Constant  Value=LowerLimit
  Discrete-Time Integrator : DiscreteIntegrator  IntegratorMethod=Integration: Trapezoidal  InitialCondition=Init  SampleTime=Ts  LimitOutput=on  UpperSaturationLimit=UpperLimit  LowerSaturationLimit=LowerLimit  ShowStatePort=on  ICPrevOutput=DiscIntNeverNeededParam  ICPrevScaledInput=DiscIntNeverNeededParam
  Kp4 : Gain  Gain=Kp  SaturateOnIntegerOverflow=on  SampleTime=Ts  OutDataTypeStr=Inherit: Same as input  ParamDataTypeStr=Inherit: Same as input
  Kp5 : Gain  Gain=Ki  SaturateOnIntegerOverflow=on  SampleTime=Ts  OutDataTypeStr=Inherit: Same as input  ParamDataTypeStr=Inherit: Same as input
  Logical Operator : Logic  AllPortsSameDT=off  OutDataTypeStr=boolean
  Logical Operator1 : Logic  AllPortsSameDT=off  OutDataTypeStr=boolean
  Logical Operator2 : Logic  Operator=OR  AllPortsSameDT=off  OutDataTypeStr=boolean
  Relational Operator : RelationalOperator  OutDataTypeStr=boolean  InputSameDT=off
  Relational Operator1 : RelationalOperator  Operator=<=  OutDataTypeStr=boolean  InputSameDT=off
  Saturation2 : Saturate  UpperLimit=UpperLimit  LowerLimit=LowerLimit  SampleTime=Ts
  Sum1 : Sum  InputSameDT=on  SaturateOnIntegerOverflow=on  SampleTime=Ts  OutDataTypeStr=Inherit: Same as first input
  Sum6 : Sum  InputSameDT=on  SaturateOnIntegerOverflow=on  SampleTime=Ts  OutDataTypeStr=Inherit: Same as first input
  Switch : Switch  Criteria=u2 > Threshold  SaturateOnIntegerOverflow=off  InputSameDT=off
  Zero-Order Hold : ZeroOrderHold  SampleTime=Ts
  Out : Outport  SampleTime=Ts  InitialOutput=0
  wires:
  Kp5/1 -> Switch/3
  Switch/1 -> Discrete-Time Integrator/1
  Saturation2/1 -> Out/1
  Discrete-Time Integrator/1 -> Sum6/2
  Kp4/1 -> Zero-Order Hold/1
  Sum6/1 -> Saturation2/1
  Error/1 -> Kp5/1, Kp4/1, Compare To Zero/1, Compare To Zero1/1
  Compare To Zero1/1 -> Logical Operator1/2  "Error_is_negative"
  Logical Operator1/1 -> Logical Operator2/2
  Logical Operator/1 -> Logical Operator2/1
  Compare To Zero/1 -> Logical Operator/2  "Error_is_positive"
  Constant3/1 -> Relational Operator1/2
  Constant1/1 -> Relational Operator/2
  Relational Operator1/1 -> Logical Operator1/1  "LowerLimit_Is_Reached"
  Relational Operator/1 -> Logical Operator/1  "UpperLimit_is_Reached"
  Logical Operator2/1 -> Switch/2
  Sum1/1 -> Relational Operator/1, Relational Operator1/1
  Discrete-Time Integrator/State -> Sum1/1
  Zero-Order Hold/1 -> Sum6/1, Sum1/2
  Constant/1 -> Switch/1

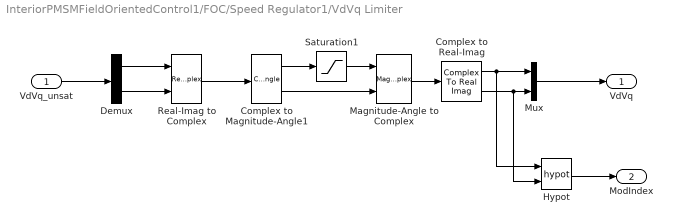
== system InteriorPMSMFieldOrientedControl1/FOC/Speed Regulator1/VdVq Limiter ==
  VdVq_unsat : Inport
  Complex to Magnitude-Angle1 : ComplexToMagnitudeAngle
  Complex to Real-Imag : ComplexToRealImag
  Demux : Demux  Outputs=2
  Hypot : Math  Operator=hypot
  Magnitude-Angle to Complex : MagnitudeAngleToComplex
  Mux : Mux  Inputs=2
  Real-Imag to Complex : RealImagToComplex
  Saturation1 : Saturate  UpperLimit=2/sqrt(3)  LowerLimit=0
  VdVq : Outport
  ModIndex : Outport  Port=2
  wires:
  Real-Imag to Complex/1 -> Complex to Magnitude-Angle1/1
  Saturation1/1 -> Magnitude-Angle to Complex/1
  Complex to Magnitude-Angle1/2 -> Magnitude-Angle to Complex/2
  Complex to Magnitude-Angle1/1 -> Saturation1/1
  Magnitude-Angle to Complex/1 -> Complex to Real-Imag/1
  Demux/1 -> Real-Imag to Complex/1
  Demux/2 -> Real-Imag to Complex/2
  VdVq_unsat/1 -> Demux/1
  Complex to Real-Imag/1 -> Hypot/1, Mux/1
  Complex to Real-Imag/2 -> Hypot/2, Mux/2
  Mux/1 -> VdVq/1
  Hypot/1 -> ModIndex/1

== matlab function InteriorPMSMFieldOrientedControl1/FOC/Current reference calculation/MTPA Field Weakening Controller ==
  data: iqn_opt input; Ten input; iqn output; w input; Vdc input; params input; idn output
function [iqn,idn] = fcn(iqn_opt,Ten,w,Vdc,params)
% Maximum Torque Per Ampere (MTPA) Field Weakening Controller
% Olivier Tremblay, ETS 2008

kFact = 0.92; % safety factor 
Ld = params(1); % Ld inductance (H)
Lq = params(2); % Lq inductance (H)
lam = params(3); % Flux induced by magnets (Wb)
p = params(4); % Number of poles pairs
ib = params(5); % Base current
% Vs = Vdc/(pi/2)*kFact;  % Maximum operation with hysteresis modulation
Vs = Vdc/(sqrt(3))*kFact;  % Maximum operation with PWM 
ten = abs(Ten); %Normalized required torque
iqn = sign(Ten)*iqn_opt; %Normalized required q optimal current

if Ten == 0 && w == 0 % No speed and required torque = 0
    idn = 0;
elseif iqn ~= 0 % Normal operation, idn is a function of Ten and iqn
    idn = 1-Ten/iqn;
else %Special case if iqn = 0. To avoid zero division we calculate the current required to maintain speed
    idn = -(lam*p*w-Vs*kFact)/(p*Ld*w*ib);
end

%Overspeed: field weakening mode
if sqrt((-Lq*p*w*iqn*ib)^2+(Ld*p*w*idn*ib+lam*p*w)^2) >= Vs 
    vs = Vs;
    k1 = 2*lam*Ld/(ib*Lq^2);
    k2 = Ld^2/Lq^2;
    k3 = lam^2/(ib^2*Lq^2)+k2;
    
    g2 = -vs^2/(p^2*ib^2*Lq^2*w^2) + k1 + k3;
    g3 = -k1*ten-2*ten*k2;
    g4 = k2*ten^2;
    
    a1 = abs(-768*g4^3+384*g4^2*g2^2-48*g4*g2^4-432*g2*g4*g3^2+81*g3^4+12*g3^2*g2^3)^(1/2);
    a2 = (-288*g2*g4+108*g3^2+8*g2^3+12*a1)^(1/3);
    a3 = (-4*g2+a2+48/a2*g4+4/a2*g2^2)^(1/2);
    iqn = (1/12*6^(1/2)*a3+1/12*abs(-48*g2-6*a2-288/a2*g4-24/a2*g2^2-72/a3*g3*6^(1/2))^(1/2));
    iqn = sign(Ten)*iqn;

    idn = 1-Ten/iqn;
end

== matlab function InteriorPMSMFieldOrientedControl1/SVPWM Modulator/MATLAB Function ==
  data: Ts parameter; Fsw parameter; Vref input; P output; PWMmethod parameter; D output; Clk input; Pavg parameter
function [P, D]   = ...
    UnifiedPWMModulator_2Levelx(Ts, Fsw, Vref, PWMmethod, Clk, Pavg)
[P, D]   = ...
    UnifiedPWMModulator2Level(Ts, Fsw, Vref, PWMmethod, Pavg, Clk);
